simulink model "NL_function_block"  (R2024b)
settings: Solver=VariableStepAuto  StartTime=0.0  StopTime=10.0  RelTol=1e-3
values from neighbouring files (symbols this model uses):
  X0 = [x_e; xd_e; i_e]    [NL_model.m]
settings Model: Creator=edoardo  LastModifiedBy=edoardo

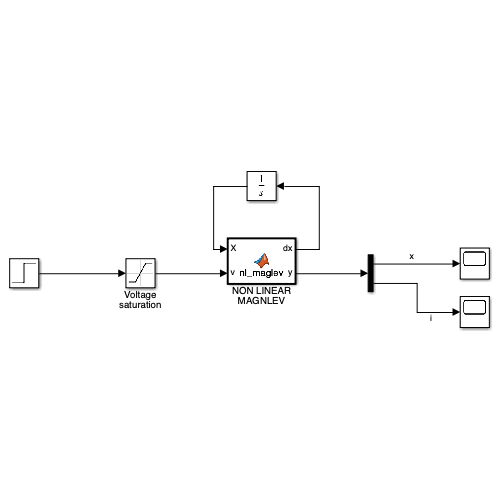
[thumbnail: Simulink's stored preview of the top-level diagram]
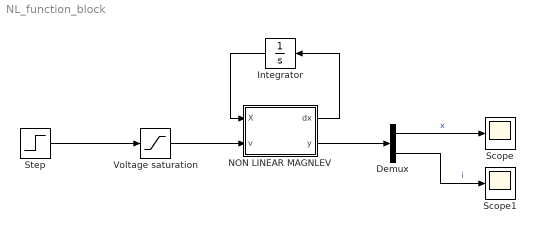
== system NL_function_block ==
  Demux : Demux  Outputs=2
  Integrator : Integrator  InitialCondition=X0
  NON LINEAR MAGNLEV : MATLAB Function  TreatAsAtomicUnit=on
  Scope : Scope
  Scope1 : Scope
  Step : Step  SampleTime=0
  Voltage saturation : Saturate  UpperLimit=3  LowerLimit=-3
  wires:
  NON LINEAR MAGNLEV/1(dx) -> Integrator/1
  Integrator/1 -> NON LINEAR MAGNLEV/1(X)
  NON LINEAR MAGNLEV/2(y) -> Demux/1
  Demux/1 -> Scope/1  "x"
  Demux/2 -> Scope1/1  "i"
  Step/1 -> Voltage saturation/1
  Voltage saturation/1 -> NON LINEAR MAGNLEV/2(v)

== matlab function NL_function_block/NON LINEAR MAGNLEV ==
  data: dx output; X input; y output; v input
function [dx, y] = nl_maglev(X, v)
% Stati:
%   X(1) = x     posizione sfera [m]
%   X(2) = xdot  velocita sfera [m/s]
%   X(3) = i     corrente bobina [A]
%
% Ingresso:
%   v = comando al VoltPAQ [V], prima del guadagno Kg
%
% Uscite:
%   y(1) = x
%   y(2) = i

dx = zeros(3,1);
y  = zeros(2,1);

%% Parametri elettrici
Kg = 3;

L = 412.5e-3;      % [H]
Rc = 10;           % [ohm]
Rs = 1;            % [ohm]
Rcal = 0.85;
R = (Rc + Rs)*Rcal;

V_max = 24;        % [V] limite tensione bobina

%% Parametri meccanici
km = 6.5308e-5;    % [N*m^2/A^2]
r = 1.27e-2;       % [m]
m = 0.068;         % [kg]
l = 0.0394;        % [m]
g = 9.81;          % [m/s^2]

%% Stati grezzi
x1_raw = X(1);     % posizione [m]
x2_raw = X(2);     % velocita [m/s]
x3     = X(3);     % corrente [A]

%% Saturazioni fisiche
x_min = 0;                         % pallina appoggiata sul post
x_max = l - 2*r;                   % circa 0.014 m, posizione massima teorica
eps_gap = 1e-4;                    % evita divisione per zero vicino al magnete

% Posizione usata nel modello
x1 = max(x1_raw, x_min);

% Saturazione superiore solo per evitare singolarità numerica
% Se vuoi davvero 0-inf, questa riga serve comunque a proteggere il denominatore.
x1_force = min(x1, x_max - eps_gap);

%% Amplificatore con saturazione di tensione
u = Kg*v;
u = min(max(u, -V_max), V_max);

%% Dinamica non lineare
gap = l - 2*r - x1_force;

x1_d_free = x2_raw;

x2_d_free = (km/m) * x3^2/(gap^2) - g;

x3_d = (u - R*x3)/L;

%% Vincolo al fine corsa inferiore
% Se la pallina è sul post e sta andando verso il basso,
% blocco la posizione a zero.
if x1_raw <= x_min && x2_raw < 0 && x2_d_free <= 0
    x1_d = 0;
    x2_d = 0;
else
    x1_d = x1_d_free;
    x2_d = x2_d_free;
end

%% Derivata dello stato
dx(1) = x1_d;
dx(2) = x2_d;
dx(3) = x3_d;

%% Uscite fisiche
y(1) = max(x1_raw, x_min);
y(2) = x3;

end
